simulink model "vibration"  (R2022b)
settings: Solver=VariableStepAuto  StartTime=0.0  StopTime=10.0  RelTol=1e-3
undefined symbols (not defined in the file or in its folder): magnitude
settings Model: Creator=integzz  LastModifiedBy=integzz

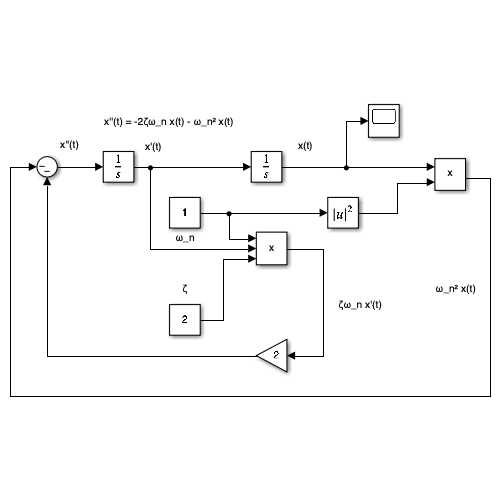
[thumbnail: Simulink's stored preview of the top-level diagram]
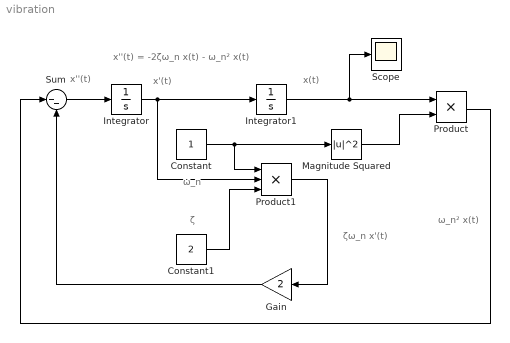
== system vibration ==
  note: x''(t) = -2ζω_n x(t) - ω_n² x(t)
  note: ζω_n x'(t)
  note: ζ
  note: ω_n
  note: ω_n² x(t)
  note: x(t)
  note: x'(t)
  note: x''(t)
  Constant : Constant
  Constant1 : Constant  Value=2
  Gain : Gain  Gain=2
  Integrator : Integrator
  Integrator1 : Integrator  InitialCondition=5
  Magnitude Squared : Math  Operator=magnitude^2
  Product : Product
  Product1 : Product  Inputs=3
  Scope : Scope
  Sum : Sum  Inputs=|--
  wires:
  Integrator/1 -> Product1/2, Integrator1/1
  Integrator1/1 -> Scope/1, Product/1
  Constant1/1 -> Product1/3
  Constant/1 -> Magnitude Squared/1, Product1/1
  Magnitude Squared/1 -> Product/2
  Sum/1 -> Integrator/1
  Product/1 -> Sum/1
  Product1/1 -> Gain/1
  Gain/1 -> Sum/2
